simulink model "EnergyEstimation_and_RobotActuation"  (R2021a)
settings: Solver=ode14x  StartTime=0.0  StopTime=10  FixedStep=.001  MaxStep=0.1  RelTol=1e-3
undefined symbols (not defined in the file): National_Instruments, PCI
libraries: sldrtlib x14
settings Model: Creator=cdm930PC_5  LastModifiedBy=cdm930PC_5
settings SolverCC: AlgebraicLoopSolver=TrustRegion
settings DataIOCC: ReturnWorkspaceOutputs=off
settings DebuggingCC: SFMachineParentedDataDiag=warning  ArithmeticOperatorsInVariantConditions=warning
settings SFSimCC: CustomCodeUndefinedFunction=UseInterfaceOnly
settings RTWCC: Description=Simulink Desktop Real-Time  SystemTargetFile=sldrt.tlc  TemplateMakefile=sldrt.tmf  RTWCompilerOptimization=on
settings CodeAppCC: MaxIdLength=95
settings SimulinkDesktopRealTimeCC: TargetPreCompLibLocation=C:\Program Files\Polyspace\R2021a\toolbox\sldrt\lib\win64

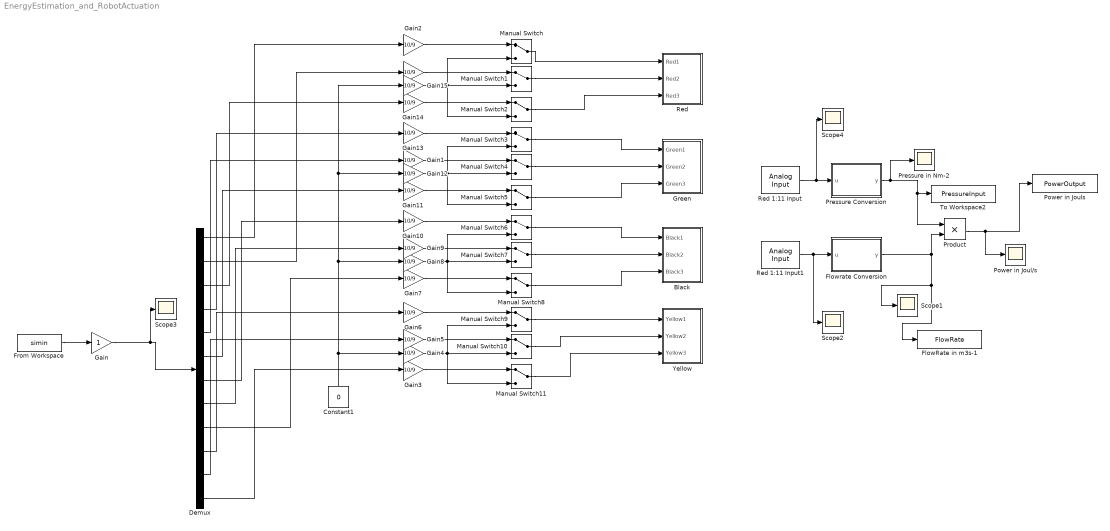
== system EnergyEstimation_and_RobotActuation ==
  " " : Gain  Gain=10/9
  Black : Subsystem
  Constant1 : Constant  Value=0
  Demux : Demux  Outputs=12
  FlowRate in m3s-1 : ToWorkspace  VariableName=FlowRate  SaveFormat=Timeseries  SampleTime=-1
  Flowrate Conversion : MATLAB Function  TreatAsAtomicUnit=on
  From Workspace : FromWorkspace  VariableName=simin
  Gain : Gain
  Gain{1..15} (15 alike) : Gain  Gain=10/9
  Green : Subsystem
  Manual Switch{,1..11} (12 alike) : ManualSwitch
  Power in Joul/s : Scope
  Power in Jouls : ToWorkspace  VariableName=PowerOutput  SaveFormat=Timeseries  SampleTime=-1
  Pressure Conversion : MATLAB Function  TreatAsAtomicUnit=on
  Pressure in Nm-2 : Scope
  Product : Product
  "Red " : Subsystem
  Red 1:11 Input : sldrtlib/Analog Input  SampleTime=0.003  MaxMissedTicks=inf  ShowMissedTicks=off  YieldWhenWaiting=on  DrvName=National_Instruments/PCI-6225  DrvAddress=4294967295  DrvOptions=[0 0 0 0 0]  Channels=1  RangeMode=1  VoltRange=1  DataType=1
      settings: AttributesFormatString=National Instruments\nPCI-6225 [auto]
  Red 1:11 Input1 : sldrtlib/Analog Input  SampleTime=0.003  MaxMissedTicks=inf  ShowMissedTicks=off  YieldWhenWaiting=on  DrvName=National_Instruments/PCI-6225  DrvAddress=4294967295  DrvOptions=[0 0 0 0 0]  Channels=2  RangeMode=1  VoltRange=1  DataType=1
      settings: AttributesFormatString=National Instruments\nPCI-6225 [auto]
  Scope{1..4} (4 alike) : Scope
  To Workspace2 : ToWorkspace  VariableName=PressureInput  SaveFormat=Timeseries  SampleTime=-1
  Yellow : Subsystem
  wires:
  Manual Switch/1 -> "Red "/1(Red1)
  Manual Switch1/1 -> "Red "/2(Red2)
  Manual Switch2/1 -> "Red "/3(Red3)
  Demux/2 -> " "/1
  Demux/3 -> Gain14/1
  Constant1/1 -> Gain15/1, Gain12/1, Gain8/1, Gain4/1
  Demux/6 -> Gain11/1
  Demux/5 -> Gain1/1
  Manual Switch5/1 -> Green/3(Green3)
  Manual Switch4/1 -> Green/2(Green2)
  Manual Switch3/1 -> Green/1(Green1)
  Demux/4 -> Gain13/1
  Demux/7 -> Gain10/1
  Manual Switch6/1 -> Black/1(Black1)
  Manual Switch7/1 -> Black/2(Black2)
  Manual Switch8/1 -> Black/3(Black3)
  Demux/8 -> Gain9/1
  Demux/9 -> Gain7/1
  Demux/12 -> Gain3/1
  Demux/11 -> Gain5/1
  Demux/10 -> Gain6/1
  Manual Switch9/1 -> Yellow/1(Yellow1)
  Manual Switch10/1 -> Yellow/2(Yellow2)
  Manual Switch11/1 -> Yellow/3(Yellow3)
  Gain2/1 -> Manual Switch/1
  Gain4/1 -> Manual Switch11/2, Manual Switch9/2, Manual Switch10/2
  Gain6/1 -> Manual Switch9/1
  Gain8/1 -> Manual Switch7/2, Manual Switch6/2, Manual Switch8/2
  Gain10/1 -> Manual Switch6/1
  Gain11/1 -> Manual Switch5/1
  Gain12/1 -> Manual Switch5/2, Manual Switch3/2, Manual Switch4/2
  Gain1/1 -> Manual Switch4/1
  Gain13/1 -> Manual Switch3/1
  Gain14/1 -> Manual Switch2/1
  Gain15/1 -> Manual Switch1/2, Manual Switch/2, Manual Switch2/2
  Demux/1 -> Gain2/1
  " "/1 -> Manual Switch1/1
  From Workspace/1 -> Gain/1
  Gain/1 -> Scope3/1, Demux/1
  Gain9/1 -> Manual Switch7/1
  Gain7/1 -> Manual Switch8/1
  Gain5/1 -> Manual Switch10/1
  Gain3/1 -> Manual Switch11/1
  Red 1:11 Input/1 -> Scope4/1, Pressure Conversion/1(u)
  Pressure Conversion/1(y) -> Product/1, To Workspace2/1, Pressure in Nm-2/1
  Flowrate Conversion/1(y) -> FlowRate in m3s-1/1, Scope1/1, Product/2
  Red 1:11 Input1/1 -> Scope2/1, Flowrate Conversion/1(u)
  Product/1 -> Power in Joul/s/1, Power in Jouls/1

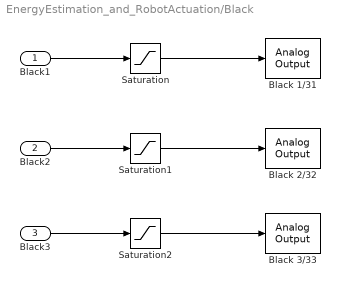
== system EnergyEstimation_and_RobotActuation/Black ==
  Black1 : Inport
  Black2 : Inport  Port=2
  Black3 : Inport  Port=3
  Black 1/31 : sldrtlib/Analog Output  SampleTime=0.02  MaxMissedTicks=inf  ShowMissedTicks=off  YieldWhenWaiting=on  DrvName=National_Instruments/PCI-6703  DrvAddress=4294967295  DrvOptions=0  Channels=7  RangeMode=1  VoltRange=1  InitialValue=[]  FinalValue=0
      settings: AttributesFormatString=National Instruments\nPCI-6703 [auto]
  Black 2/32 : sldrtlib/Analog Output  SampleTime=0.02  MaxMissedTicks=inf  ShowMissedTicks=off  YieldWhenWaiting=on  DrvName=National_Instruments/PCI-6703  DrvAddress=4294967295  DrvOptions=0  Channels=8  RangeMode=1  VoltRange=1  InitialValue=[]  FinalValue=0
      settings: AttributesFormatString=National Instruments\nPCI-6703 [auto]
  Black 3/33 : sldrtlib/Analog Output  SampleTime=0.02  MaxMissedTicks=inf  ShowMissedTicks=off  YieldWhenWaiting=on  DrvName=National_Instruments/PCI-6703  DrvAddress=4294967295  DrvOptions=0  Channels=9  RangeMode=1  VoltRange=1  InitialValue=[]  FinalValue=0
      settings: AttributesFormatString=National Instruments\nPCI-6703 [auto]
  Saturation : Saturate  UpperLimit=7  LowerLimit=0
  Saturation1 : Saturate  UpperLimit=7  LowerLimit=0
  Saturation2 : Saturate  UpperLimit=7  LowerLimit=0
  wires:
  Black3/1 -> Saturation2/1
  Black2/1 -> Saturation1/1
  Black1/1 -> Saturation/1
  Saturation/1 -> Black 1/31/1
  Saturation1/1 -> Black 2/32/1
  Saturation2/1 -> Black 3/33/1

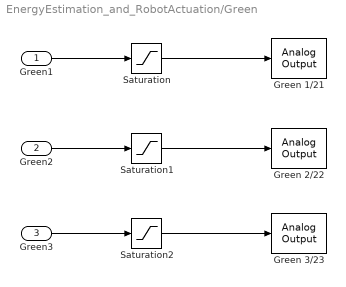
== system EnergyEstimation_and_RobotActuation/Green ==
  Green1 : Inport
  Green2 : Inport  Port=2
  Green3 : Inport  Port=3
  Green 1/21 : sldrtlib/Analog Output  SampleTime=0.02  MaxMissedTicks=inf  ShowMissedTicks=off  YieldWhenWaiting=on  DrvName=National_Instruments/PCI-6703  DrvAddress=4294967295  DrvOptions=0  Channels=4  RangeMode=1  VoltRange=1  InitialValue=[]  FinalValue=0
      settings: AttributesFormatString=National Instruments\nPCI-6703 [auto]
  Green 2/22 : sldrtlib/Analog Output  SampleTime=0.02  MaxMissedTicks=inf  ShowMissedTicks=off  YieldWhenWaiting=on  DrvName=National_Instruments/PCI-6703  DrvAddress=4294967295  DrvOptions=0  Channels=5  RangeMode=1  VoltRange=1  InitialValue=[]  FinalValue=0
      settings: AttributesFormatString=National Instruments\nPCI-6703 [auto]
  Green 3/23 : sldrtlib/Analog Output  SampleTime=0.02  MaxMissedTicks=inf  ShowMissedTicks=off  YieldWhenWaiting=on  DrvName=National_Instruments/PCI-6703  DrvAddress=4294967295  DrvOptions=0  Channels=6  RangeMode=1  VoltRange=1  InitialValue=[]  FinalValue=0
      settings: AttributesFormatString=National Instruments\nPCI-6703 [auto]
  Saturation : Saturate  UpperLimit=7  LowerLimit=0
  Saturation1 : Saturate  UpperLimit=7  LowerLimit=0
  Saturation2 : Saturate  UpperLimit=7  LowerLimit=0
  wires:
  Green1/1 -> Saturation/1
  Green3/1 -> Saturation2/1
  Green2/1 -> Saturation1/1
  Saturation/1 -> Green 1/21/1
  Saturation1/1 -> Green 2/22/1
  Saturation2/1 -> Green 3/23/1

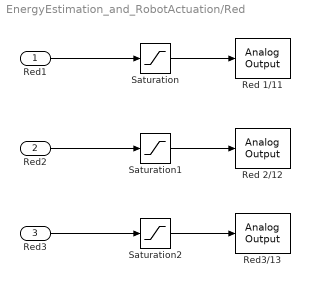
== system EnergyEstimation_and_RobotActuation/Red  ==
  Red1 : Inport
  Red2 : Inport  Port=2
  Red3 : Inport  Port=3
  Red 1/11 : sldrtlib/Analog Output  SampleTime=0.02  MaxMissedTicks=inf  ShowMissedTicks=off  YieldWhenWaiting=on  DrvName=National_Instruments/PCI-6703  DrvAddress=4294967295  DrvOptions=0  Channels=1  RangeMode=1  VoltRange=1  InitialValue=0  FinalValue=0
      settings: AttributesFormatString=National Instruments\nPCI-6703 [auto]
  Red 2/12 : sldrtlib/Analog Output  SampleTime=0.02  MaxMissedTicks=inf  ShowMissedTicks=off  YieldWhenWaiting=on  DrvName=National_Instruments/PCI-6703  DrvAddress=4294967295  DrvOptions=0  Channels=2  RangeMode=1  VoltRange=1  InitialValue=0  FinalValue=0
      settings: AttributesFormatString=National Instruments\nPCI-6703 [auto]
  Red3/13 : sldrtlib/Analog Output  SampleTime=0.02  MaxMissedTicks=inf  ShowMissedTicks=off  YieldWhenWaiting=on  DrvName=National_Instruments/PCI-6703  DrvAddress=4294967295  DrvOptions=0  Channels=3  RangeMode=1  VoltRange=1  InitialValue=0  FinalValue=0
      settings: AttributesFormatString=National Instruments\nPCI-6703 [auto]
  Saturation : Saturate  UpperLimit=7  LowerLimit=0
  Saturation1 : Saturate  UpperLimit=7  LowerLimit=0
  Saturation2 : Saturate  UpperLimit=7  LowerLimit=0
  wires:
  Red1/1 -> Saturation/1
  Saturation/1 -> Red 1/11/1
  Saturation1/1 -> Red 2/12/1
  Saturation2/1 -> Red3/13/1
  Red2/1 -> Saturation1/1
  Red3/1 -> Saturation2/1

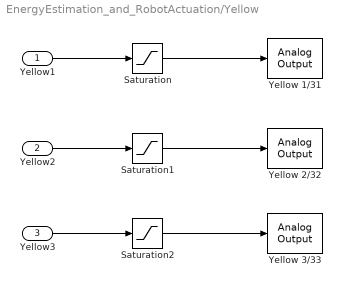
== system EnergyEstimation_and_RobotActuation/Yellow ==
  Yellow1 : Inport
  Yellow2 : Inport  Port=2
  Yellow3 : Inport  Port=3
  Saturation : Saturate  UpperLimit=5  LowerLimit=0
  Saturation1 : Saturate  UpperLimit=5  LowerLimit=0
  Saturation2 : Saturate  UpperLimit=5  LowerLimit=0
  Yellow 1/31 : sldrtlib/Analog Output  SampleTime=0.02  MaxMissedTicks=inf  ShowMissedTicks=off  YieldWhenWaiting=on  DrvName=National_Instruments/PCI-6703  DrvAddress=4294967295  DrvOptions=0  Channels=10  RangeMode=1  VoltRange=1  InitialValue=[]  FinalValue=0
      settings: AttributesFormatString=National Instruments\nPCI-6703 [auto]
  Yellow 2/32 : sldrtlib/Analog Output  SampleTime=0.02  MaxMissedTicks=inf  ShowMissedTicks=off  YieldWhenWaiting=on  DrvName=National_Instruments/PCI-6703  DrvAddress=4294967295  DrvOptions=0  Channels=11  RangeMode=1  VoltRange=1  InitialValue=[]  FinalValue=0
      settings: AttributesFormatString=National Instruments\nPCI-6703 [auto]
  Yellow 3/33 : sldrtlib/Analog Output  SampleTime=0.02  MaxMissedTicks=inf  ShowMissedTicks=off  YieldWhenWaiting=on  DrvName=National_Instruments/PCI-6703  DrvAddress=4294967295  DrvOptions=0  Channels=12  RangeMode=1  VoltRange=1  InitialValue=[]  FinalValue=0
      settings: AttributesFormatString=National Instruments\nPCI-6703 [auto]
  wires:
  Saturation2/1 -> Yellow 3/33/1
  Saturation1/1 -> Yellow 2/32/1
  Saturation/1 -> Yellow 1/31/1
  Yellow1/1 -> Saturation/1
  Yellow2/1 -> Saturation1/1
  Yellow3/1 -> Saturation2/1

== matlab function EnergyEstimation_and_RobotActuation/Pressure Conversion ==
  data: u input; y output
function y = fcn(u)

y = ((u-1)/0.4)*1e5;

== matlab function EnergyEstimation_and_RobotActuation/Flowrate Conversion ==
  data: u input; y output
function y = fcn(u)

y = ((u-1)*25/4)*1.6667e-5;
